simulink model "vehicle_state_space_model_yaw_control"  (R2021b)
settings: Solver=FixedStepAuto  StartTime=0.0  StopTime=10  FixedStep=1e-03  RelTol=1e-3
undefined symbols (not defined in the file): A, B, K, sigbuilder_block
settings Model: Creator=Vishal kain  LastModifiedBy=Ronak Jain
settings DataIOCC: SaveState=on
settings DebuggingCC: UnderSpecifiedDimensionMsg=warning

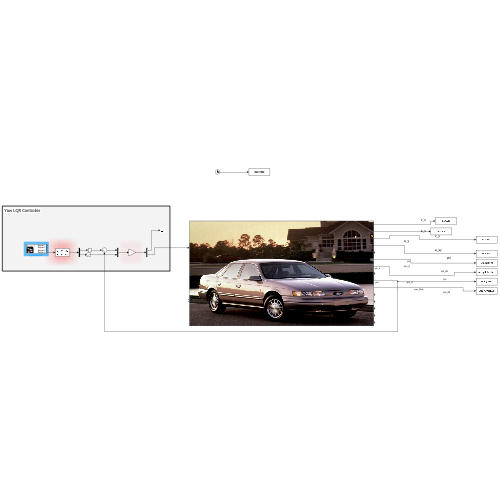
[thumbnail: Simulink's stored preview of the top-level diagram]
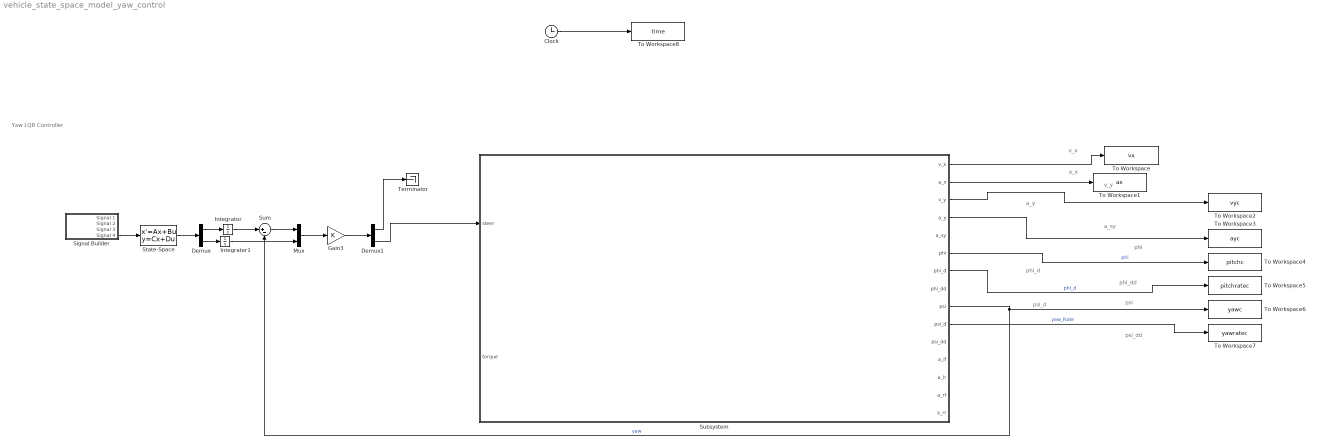
== system vehicle_state_space_model_yaw_control ==
  note: Yaw LQR Controller
  note: psi_dd
  note: psi_d
  note: psi
  note: phi_dd
  note: phi_d
  note: a_x
  note: v_x
  note: v_y
  note: a_y
  note: a_sy
  note: phi
  Clock : Clock
  Demux : Demux  Outputs=2
  Demux1 : Demux  Outputs=2
  Gain3 : Gain  Gain=K
  Integrator : Integrator
  Integrator1 : Integrator
  Mux : Mux  Inputs=2
  Signal Builder : Subsystem  Tag=STV Subsys  LoadFcn=sigbuilder_block('load',[5.4 36 1141.2 516.6 ]);  StartFcn=sigbuilder_block('start');  StopFcn=sigbuilder_block('stop');  ClipboardFcn=sigbuilder_block('clipboard');  mask(Sigbuilder block){tuvar=[0:10]}
      mask help: Simulink:masks:SigbuilderBlock_MD
      mask init:
      | if ~strcmp(get_param(bdroot(gcbh),'SimulationStatus'),'stopped') tuvar = sigbuilder_block('maskInit'); end
      settings: CopyFcn=sigbuilder_block('copy');  DeleteFcn=sigbuilder_block('delete');  ModelCloseFcn=sigbuilder_block('modelClose');  PreSaveFcn=sigbuilder_block('preSave');  PauseFcn=sigbuilder_block('pause');  ContinueFcn=sigbuilder_block('continue');  NameChangeFcn=sigbuilder_block('namechange');  OpenFcn=sigbuilder_block('open',[5.4 36 1141.2 516.6 ]);  CloseFcn=sigbuilder_block('close');
      mask Display: plot(0, 0, 100, 100,[2, 2, 32, 32, 2], [68, 8, 8, 68, 68],[32, 2], [38, 38], [32, 19, 2],[53, 60, 44], [32, 17, 17, 2],[16, 16, 31, 31]);txt = getActiveGroup(gcbh);text(2, 100, txt,'verticalAlignment', 'top');
  State-Space : StateSpace  A=A  B=B  C=[1 0;0 1]  D=[0;0]  InitialCondition=0
  Subsystem : Subsystem
      mask Display: image('ford taurus.jpg'); % Use "Edit Image" on toolstrip to change.
  Sum : Sum  Inputs=|+-
  Terminator : Terminator
  To Workspace : ToWorkspace  VariableName=vx  SaveFormat=Timeseries  SampleTime=-1
  To Workspace1 : ToWorkspace  VariableName=ax  SaveFormat=Timeseries  SampleTime=-1
  To Workspace2 : ToWorkspace  VariableName=vyc  SaveFormat=Timeseries  SampleTime=-1
  To Workspace3 : ToWorkspace  VariableName=ayc  SaveFormat=Timeseries  SampleTime=-1
  To Workspace4 : ToWorkspace  VariableName=pitchc  SaveFormat=Timeseries  SampleTime=-1
  To Workspace5 : ToWorkspace  VariableName=pitchratec  SaveFormat=Timeseries  SampleTime=-1
  To Workspace6 : ToWorkspace  VariableName=yawc  SaveFormat=Timeseries  SampleTime=-1
  To Workspace7 : ToWorkspace  VariableName=yawratec  SaveFormat=Timeseries  SampleTime=-1
  To Workspace8 : ToWorkspace  VariableName=time  SaveFormat=Timeseries  SampleTime=-1
  wires:
  Subsystem/9(psi) -> Sum/2, To Workspace6/1  "yaw"
  Subsystem/10(psi_d) -> To Workspace7/1  "yaw_Rate"
  State-Space/1 -> Demux/1
  Demux/2 -> Integrator1/1
  Demux/1 -> Integrator/1
  Integrator1/1 -> Mux/2
  Mux/1 -> Gain3/1
  Gain3/1 -> Demux1/1
  Integrator/1 -> Sum/1
  Sum/1 -> Mux/1
  Demux1/2 -> Subsystem/1(steer)
  Subsystem/6(phi) -> To Workspace4/1  "phi"
  Subsystem/7(phi_d) -> To Workspace5/1  "phi_d"
  Signal Builder/4(Signal 4) -> State-Space/1
  Subsystem/1(v_x) -> To Workspace/1
  Subsystem/2(a_x) -> To Workspace1/1
  Subsystem/3(v_y) -> To Workspace2/1
  Subsystem/4(a_y) -> To Workspace3/1
  Clock/1 -> To Workspace8/1
  Demux1/1 -> Terminator/1

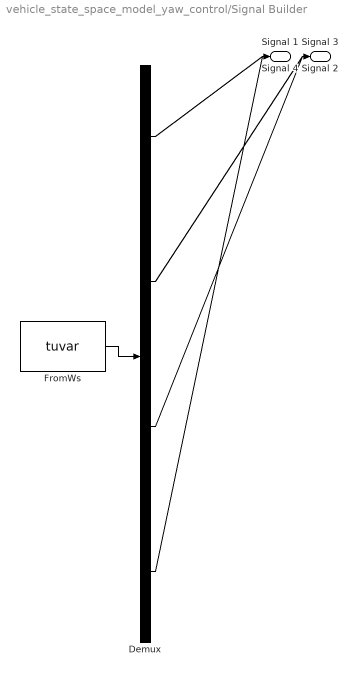
== system vehicle_state_space_model_yaw_control/Signal Builder ==
  Demux : Demux  Tag=STV Demux
      settings: DisplayOption=none
  FromWs : FromWorkspace  Tag=STV FromWs  VariableName=tuvar
      SigBuilderData=|
      | common.afterFinalStr = 'Extrapolate'
      | common.sampleTime = 0
      | dataSet.timeRange = [0 10]
      | dataSet.name = 'Group 1'
      | sbobj.Groups.Name = 'Group 1'
      | sbobj.Groups.Signals(1).Name = 'Signal 1'
      | sbobj.Groups.Signals(1).XData = [0 4 4 6 6 10]
      | sbobj.Groups.Signals(1).YData = [0 0.125 1 1 0 0]
      | sbobj.Groups.Signals(2).Name = 'Signal 2'
      | sbobj.Groups.Signals(2).XData = [0 10]
      | sbobj.Groups.Signals(2).YData = [1 1]
      | sbobj.Groups.Signals(3).Name = 'Signal 3'
      | sbobj.Groups.Signals(3).XData = [0 0.125 0.25 0.375 0.5 0.625 0.75 0.875 1 1.125 1.25 1.375 1.5 1.625 1.75 1.875 2 2.125 2.25 2.375 2.5 2.625 2.75 2.875 3 3.125 3.25 3.375 3.5 3.625 3.75 3.875 4 4.125 4.25 4.375 4.5 4.625 4.75 4.875 5 5.125 5.25 5.375 5.5 5.625 5.75 5.875 6 6.125 6.25 6.375 6.5 6.625 6.75 6.875 7 7.125 7.25 7.375 7.5 7.625 7.75 7.875 8 8.125 8.25 8.375 8.5 8.625 8.75 8.875 9 9.125 9.25 9.375 9.5 9.625 9.75 9.875 10]
      | sbobj.Groups.Signals(3).YData = [1 29.2842712475 41 29.2842712475 1 -27.2842712475 -39 -27.2842712475 1 29.2842712475 41 29.2842712475 1 -27.2842712475 -39 -27.2842712475 1 29.2842712475 41 29.2842712475 1 -27.2842712475 -39 -27.2842712475 1 29.2842712475 41 29.2842712475 1 -27.2842712475 -39 -27.2842712475 1 29.2842712475 41 29.2842712475 1 -27.2842712475 -39 -27.2842712475 1 29.2842712475 41 29.2842712475 1 -27.2842712475 -39 -27.2842712475 1 29.2842712475 41 29.2842712475 1 -27.2842712475 -39 -27.2842712475 1 29.2842712475 41 29.2842712475 1 -27.2842712475 -39 -27.2842712475 1 29.2842712475 41 29.2842712475 1 -27.2842712475 -39 -27.2842712475 1 29.2842712475 41 29.2842712475 1 -27.2842712475 -39 -27.2842712475 1]
      | sbobj.Groups.Signals(4).Name = 'Signal 4'
      | sbobj.Groups.Signals(4).XData = [0 1.25 2.5 3.75 5 6.25 7.5 8.75 10]
      | sbobj.Groups.Signals(4).YData = [1 29.2842712475 41 29.2842712475 1 -27.2842712475 -27 -27.2842712475 1]
  Signal 1 : Outport  Tag=STV Outport
  Signal 2 : Outport  Tag=STV Outport  Port=2
  Signal 3 : Outport  Tag=STV Outport  Port=3
  Signal 4 : Outport  Tag=STV Outport  Port=4
  wires:
  FromWs/1 -> Demux/1
  Demux/1 -> Signal 1/1
  Demux/2 -> Signal 2/1
  Demux/3 -> Signal 3/1
  Demux/4 -> Signal 4/1

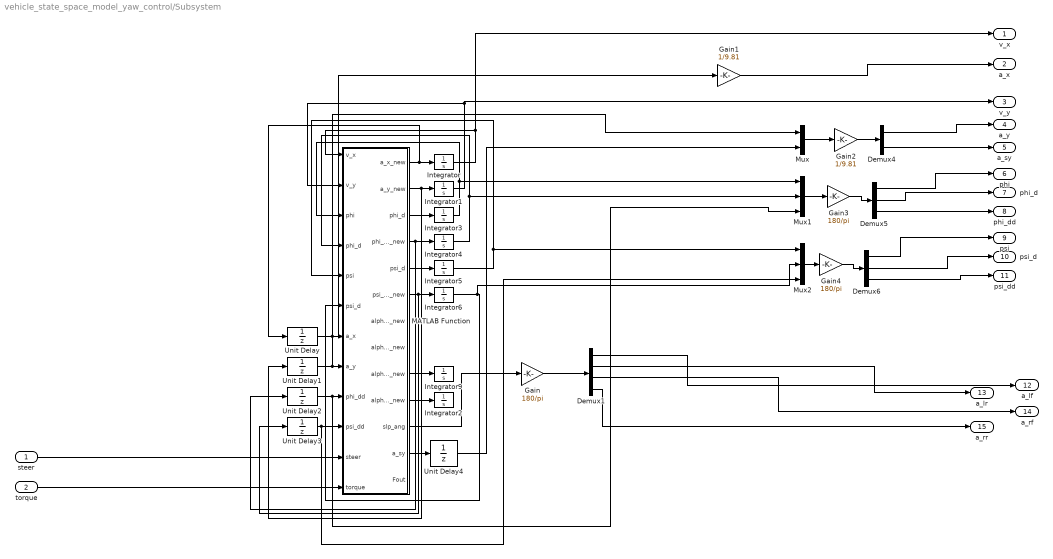
== system vehicle_state_space_model_yaw_control/Subsystem ==
  steer : Inport
  torque : Inport  Port=2
  Demux1 : Demux
  Demux4 : Demux  Outputs=2
  Demux5 : Demux  Outputs=3
  Demux6 : Demux  Outputs=3
  Gain : Gain  Gain=180/pi
  Gain1 : Gain  Gain=1/9.81
  Gain2 : Gain  Gain=1/9.81
  Gain3 : Gain  Gain=180/pi
  Gain4 : Gain  Gain=180/pi
  Integrator{,1..6,9} (8 alike) : Integrator  InitialCondition=0.0001
  MATLAB Function : MATLAB Function  TreatAsAtomicUnit=on
  Mux : Mux  Inputs=2
  Mux1 : Mux  Inputs=3
  Mux2 : Mux  Inputs=3
  Unit Delay{,1..4} (5 alike) : UnitDelay  SampleTime=-1  HasFrameUpgradeWarning=on
  v_x : Outport
  a_x : Outport  Port=2
  v_y : Outport  Port=3
  a_y : Outport  Port=4
  a_sy : Outport  Port=5
  phi : Outport  Port=6
  phi_d : Outport  Port=7
  phi_dd : Outport  Port=8
  psi : Outport  Port=9
  psi_d : Outport  Port=10
  psi_dd : Outport  Port=11
  a_lf : Outport  Port=12
  a_lr : Outport  Port=13
  a_rf : Outport  Port=14
  a_rr : Outport  Port=15
  wires:
  Mux2/1 -> Gain4/1
  Unit Delay1/1 -> Mux/1, MATLAB Function/8(a_y)
  Integrator5/1 -> MATLAB Function/5(psi), Mux2/1
  torque/1 -> MATLAB Function/12(torque)
  Integrator3/1 -> Mux1/1, MATLAB Function/3(phi)
  Demux6/3 -> psi_dd/1
  Unit Delay3/1 -> Mux2/3, MATLAB Function/10(psi_dd)
  Integrator4/1 -> Mux1/2, MATLAB Function/4("phi_d ")
  Integrator6/1 -> Mux2/2, MATLAB Function/6("psi_d ")
  Gain3/1 -> Demux5/1
  MATLAB Function/6(psi_dd_new) -> Unit Delay3/1, Integrator6/1
  Gain4/1 -> Demux6/1
  Unit Delay4/1 -> Mux/2
  Integrator/1 -> v_x/1, MATLAB Function/1(v_x)
  Integrator1/1 -> v_y/1, MATLAB Function/2(v_y)
  Demux5/2 -> phi_d/1
  Demux4/2 -> a_sy/1
  Unit Delay/1 -> Gain1/1, MATLAB Function/7(a_x)
  Unit Delay2/1 -> Mux1/3, MATLAB Function/9(phi_dd)
  MATLAB Function/10(alpha_rr_new) -> Integrator2/1
  Mux1/1 -> Gain3/1
  Gain2/1 -> Demux4/1
  MATLAB Function/4(phi_dd_new) -> Unit Delay2/1, Integrator4/1
  MATLAB Function/9(alpha_rf_new) -> Integrator9/1
  MATLAB Function/2(a_y_new) -> Unit Delay1/1, Integrator1/1
  MATLAB Function/3(phi_d) -> Integrator3/1
  Demux1/1 -> a_lf/1
  Mux/1 -> Gain2/1
  MATLAB Function/5(psi_d) -> Integrator5/1
  Demux1/2 -> a_lr/1
  Gain/1 -> Demux1/1
  MATLAB Function/1(a_x_new) -> Unit Delay/1, Integrator/1
  MATLAB Function/11(slp_ang) -> Gain/1
  MATLAB Function/12(a_sy) -> Unit Delay4/1
  Gain1/1 -> a_x/1
  Demux1/3 -> a_rf/1
  steer/1 -> MATLAB Function/11(steer)
  Demux4/1 -> a_y/1
  Demux1/4 -> a_rr/1
  Demux5/3 -> phi_dd/1
  Demux5/1 -> phi/1
  Demux6/1 -> psi/1
  Demux6/2 -> psi_d/1

== matlab function vehicle_state_space_model_yaw_control/Subsystem/MATLAB Function ==
  data: a_x_new output; a_y_new output; phi_d output; phi_dd_new output; psi_d output; psi_dd_new output; alpha_lf_new output; alpha_lr_new output; alpha_rf_new output; alpha_rr_new output; slp_ang output; a_sy output; v_x input; v_y input; phi input; phi_d input; psi input; psi_d input; a_x input; a_y input; phi_dd input; psi_dd input; steer input; torque input; Fout output
function [a_x_new, a_y_new, phi_d, phi_dd_new, psi_d, psi_dd_new, alpha_lf_new, alpha_lr_new, alpha_rf_new, alpha_rr_new,slp_ang,a_sy,Fout] =...
    fcn(v_x, v_y,phi, phi_d,psi,psi_d,a_x,a_y,phi_dd,psi_dd,steer,torque)
%==output==%
% output = zeros(10,1);
%==constants==%
g = 9.81;
%Car physical variables
l_fs = 1.01476;
l_rs = 1.67524;
t_f = 1.540;
t_r = 1.530;
h_f = 0.130;
h_r = 0.110;
h_cgs = 0.567851;
h_cguf = 0.320;
h_cgur = 0.320;
M = 1704.7;
M_uf = 98.1;
M_ur = 79.7;
I_xxs = 440.911;
I_xys = 0;
I_xzs = 7.54097;
I_yys = 2498.900;
I_yzs = 0;
I_zzs = 2619.28;
I_zzuf = M_uf*(t_f/2)^2;
I_zzur = M_ur*(t_r/2)^2;
I_tlf = 0.99;
I_trf = 0.99;
I_tlr = 0.99;
I_trr = 0.99;
%spring/dampers
K_spf = 30000; %N/mm
K_spr = 30000; %N/mm
B_f = 299.15; %N-s/mm
B_r = 299.15; %N-s/mm
%anti_roll bars
K_rf = 384.0*180/pi; %Nm/rad

K_rr = 344.4*180/pi;
%roll stiffness
K_phif = 0.766*K_spf*1000*t_f^2/2 + K_rf;%
K_phir = 0.827*K_spr*1000*t_r^2/2 + K_rr;%
K_phi = (K_phif + K_phir);
%roll damping
B_phif = 0.766*B_f*1000*t_f^2/2; %Nm-s/rad
B_phir = 0.827*B_r*1000*t_r^2/2;
B_phi = (B_phif + B_phir);
K_sr = 15.97; %steering-to-wheel angle ratio
%==calculated parameters==%
L = l_fs + l_rs;
M_s = M - M_uf - M_ur;
l_cgs = (M_ur*l_rs - M_uf*l_fs)/M;
l_f = l_fs + l_cgs;
l_r = l_rs - l_cgs;
M_f = M*l_r/L;
M_r = M*l_f/L;
h_o = h_f + l_f*(h_r - h_f)/L;
h_s = h_cgs - h_o;
h_uf = h_cguf - h_o;
h_ur = h_cgur - h_o;
h_cg = (M_s*h_cgs + M_uf*h_cguf + M_ur*h_cgur)/M;
%----------------------------%
%==tire properties==%
varx = [... 
    0.0, 0.0;... 
    0.1, 0.6;... 
    0.15, 0.85;... 
    1.0, 0.4]; %slip curve coordinates (slip-%, mu)
vary = [... 
    0.0, 0.0;... 
    0.08, 0.4;... 
    0.15, 0.6;... 
    0.3, 0.8;... 
    1.0, 0.4]; %slip curve coordinates (slip-%, mu)
varM = [... 
    0.0, 0.0;...
    0.1, 0.0005;...
    0.3, 0.00025;... 
    1.0, 0.0]; %slip angle (slip-angle, Moment-arm)
%tire properties
t_wid = 0.175;
t_rad = 0.292;
t_pressure = 275000;
%---------------------%
%==steering inputs==%
d_steer = steer;
%-------------------%
%==calculate internal accelerations==%
a_sx = a_x ...
    - psi_d*v_y ...
    - 2*h_s*phi_d*psi_d*cos(phi) ...
    - l_cgs*psi_d^2;
a_sy = psi_d*v_x + l_cgs*psi_dd + h_s*cos(phi)*phi_dd - h_s*phi_d^2*sin(phi) - h_s*psi_d^2*sin(phi);
a_ufx = a_x - l_f*psi_d^2;
a_ufy = a_y + l_f*psi_dd;
a_urx = a_x + l_r*psi_d^2;
a_ury = a_y - l_r*psi_dd;
%-------------------------------------%
%==rotation Matrix==%
ROT = [1,0,0; 
    0,cos(phi),sin(phi); 
    0,-sin(phi),cos(phi)];
I_b = [I_xxs+M_s*h_s^2,I_xys,I_xzs+M_s*h_s*l_cgs;... 
    I_xys,I_yys+M_s*(h_s^2+l_cgs^2),I_yzs;... 
    I_xzs+M_s*h_s*l_cgs,I_yzs,I_zzs+M_s*l_cgs^2];
I_c = ROT*I_b*ROT'; 
I_zzus = M_uf*l_f^2 + ... 
    M_ur*l_r^2 + ... 
    I_zzuf + I_zzur;
I_xxo = I_c(1,1);
I_zzo = I_c(3,3) + I_zzus; %effective I_zz
%---------------------------------------------%
%==Dynamic Weight Transfer Forces==%
Fzax = (M_s*h_s*a_sx + M_uf*h_uf*a_ufx + M_ur*h_ur*a_urx)/(2*L);
Fzayf = 1/t_f*(M_s*l_r*h_f/L*a_sy + M_uf*h_uf*a_ufy);
Fzayr = 1/t_r*(M_s*l_f*h_r/L*a_sy + M_ur*h_ur*a_ury);
Fzphif = -1/t_f*(K_phif*phi + B_phif*phi_d);
Fzphir = -1/t_r*(K_phir*phi + B_phir*phi_d);
%----------------------------------%
%==Tire Normal Forces==%
Fzlf = M*g*l_r/(2*L) - Fzax - Fzayf + Fzphif;
Fzrf = M*g*l_r/(2*L) - Fzax + Fzayf - Fzphif;
Fzlr = M*g*l_f/(2*L) + Fzax - Fzayr + Fzphir;
Fzrr = M*g*l_f/(2*L) + Fzax + Fzayr - Fzphir;
%----------------------%
%==Tire Longitudinal/Lateral Forces==%
%left front wheel velocity
v_xlf = v_x + psi_d*t_f/2;
v_ylf = v_y + psi_d*l_f;
%right front wheel velocity
v_xrf = v_x - psi_d*t_f/2;
v_yrf = v_y + psi_d*l_f;
%left rear wheel velocity
v_xlr = v_x + psi_d*t_r/2;
v_ylr = v_y - psi_d*l_r;
%right rear wheel velocity
v_xrr = v_x - psi_d*t_r/2;
v_yrr = v_y - psi_d*l_r;
%tire updates
omega_lf = (v_xlf^2 + v_ylf^2)^(1/2);
omega_rf = (v_xrf^2 + v_yrf^2)^(1/2);
omega_lr = (v_xlr^2 + v_ylr^2)^(1/2);
omega_rr = (v_xrr^2 + v_yrr^2)^(1/2);
%==Linear Cruise Control=%
if v_x < 11.1
    if omega_lf > omega_rf
        Mtlf = (11.1 - v_x)*200;
        Mtrf = 0;
    else
        Mtlf = 0;
        Mtrf = (11.1 - v_x)*200;
    end
else
    Mtlf = 0;
    Mtrf = 0;
end
Mtlf = 0;
Mtrf = 0;
Mtlr = 0;
Mtrr = 0;
%-------------------------%
%get steering angle
delta = d_steer/(180*K_sr)*pi; %radians
beta = atan(v_y/v_x);
beta_lf = atan(v_ylf/v_xlf);
beta_rf = atan(v_yrf/v_xrf);
beta_lr = atan(v_ylr/v_xlr);
beta_rr = atan(v_yrr/v_xrr);
%Interpolate forces
%Linearized Force Coefficients (C_alpha)
C_alf = vary(2,2)/vary(2,1)*Fzlf;
C_arf = vary(2,2)/vary(2,1)*Fzrf;
C_alr = vary(2,2)/vary(2,1)*Fzlr;
C_arr = vary(2,2)/vary(2,1)*Fzrr;
a_lf = beta_lf - delta;
a_rf = beta_rf - delta;
a_lr = beta_lr;
a_rr = beta_rr;
slp_ang = [a_lf,a_rf,a_lr,a_rr];
%Linear Cruise Control for constant v_x
if v_x < 11.1
    Fxtf = (11.1-v_x)*20000;
else
    Fxtf = 0; %no torque
end
Fxtlf = 0;
Fxtrf = 0;
Fxtlr = 0;
Fxtrr = 0;
Fytlf = -a_lf*C_alf;
Fytrf = -a_rf*C_arf;
Fytlr = -a_lr*C_alr;
Fytrr = -a_rr*C_arr;
Fxlf = Fxtlf*cos(delta) - Fytlf*sin(delta);
Fxrf = Fxtrf*cos(delta) - Fytrf*sin(delta);
Fxlr = Fxtlr;
Fxrr = Fxtrr;
Fylf = Fytlf*cos(delta) + Fxtlf*sin(delta);
Fyrf = Fytrf*cos(delta) + Fxtrf*sin(delta);
Fylr = Fytlr;
Fyrr = Fytrr;
Fout = [Fylf,Fyrf,Fylr,Fyrr];
Mzlf = 0;
Mzrf = 0;
Mzlr = 0;
Mzrr = 0;
%---------------------------------------%
%Omeaga/Alpha of Wheels
alpha_lf_new = (Fxtlf*t_rad + Mtlf)/I_tlf;
alpha_rf_new = (Fxtrf*t_rad + Mtrf)/I_trf;
alpha_lr_new = (Fxtlr*t_rad + Mtlr)/I_tlr;
alpha_rr_new = (Fxtrr*t_rad + Mtrr)/I_trr;
% alpha_lf_new = 0;
% alpha_rf_new = 0;
% alpha_lr_new = 0;
% alpha_rr_new = 0;
%==Torques==%
T_phif = -K_phif*phi - B_phif*phi_d;
T_phir = -K_phir*phi - B_phir*phi_d;
%-----------%
%==Sum forces and torques==%
sigFx = Fxlf + Fxrf + Fxlr + Fxrr;
sigFy = Fylf + Fyrf + Fylr + Fyrr;
sigTxs = T_phif + T_phir - ... 
    M_s*g*h_s*sin(phi) + M_s*h_s*a_sy*cos(phi);
sigTz = (Fylf + Fyrf)*l_f - (Fylr + Fyrr)*l_r + ... 
    t_f/2*(Fxlf - Fxrf) + t_r/2*(Fxlr - Fxrr) + ... 
    Mzlf + Mzrf + Mzlr + Mzrr;
%--------------------------%
%==Update independent variables==%
a_x_new = (sigFx + ... 
    M_s.*(-2*h_s.*phi_d.*psi_d.*cos(phi) - ... 
    h_s.*psi_dd.*sin(phi)))./M;
a_y_new = (sigFy - ... 
    M_s*(-h_s*phi_dd*cos(phi) + ... 
    h_s*phi_d^2*sin(phi) + ... 
    h_s*psi_d^2*sin(phi)))./M;
phi_dd_new = (sigTxs - ... 
    (I_xzs+M_s*h_s*l_cgs)*cos(phi)*psi_dd + ... 
    (I_xzs+M_s*h_s*l_cgs)*sin(phi)*phi_d*psi_d + ... 
    (I_zzs - I_yys - M_s*h_s^2)*sin(phi)*cos(phi)*psi_d^2)./ ... 
    (I_xxs+M_s*h_s^2);
psi_dd_new = (sigTz - ... 
    (I_xzs+M_s*h_s*l_cgs)*cos(phi)*phi_dd - ... 
    (I_xzs+M_s*h_s*l_cgs)*sin(phi)*phi_d^2 - ... 
    M_s*h_s*a_x*sin(phi) - ... 
    (I_zzs - I_yys - M_s*h_s^2)*sin(phi)*cos(phi)*psi_d*phi_d)./I_zzo;
%acceleration outputs
acc_out = [a_x_new,a_y_new,a_sy,phi_dd_new,psi_dd_new];
%X



end
%SPRUNG BODY
%----------------------------------%
%end
%nd
%d
%
